simulink model "Bicycle_model"  (R2020a)
settings: Solver=VariableStepAuto  StartTime=0.0  StopTime=10.0  RelTol=1e-3
settings Model: Creator=yafta  LastModifiedBy=yafta

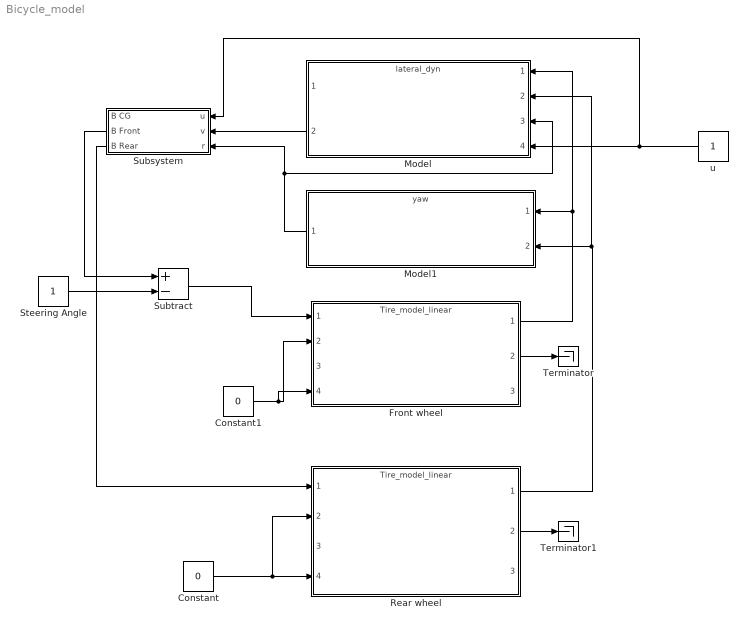
== system Bicycle_model ==
  Constant : Constant  Value=0
  Constant1 : Constant  Value=0
  Front wheel : ModelReference  ModelNameDialog=Tire_model_linear  SimulationMode=Normal  ModelReferenceVersion=1.2
  Model : ModelReference  ModelNameDialog=lateral_dyn.slx  SimulationMode=Normal  ModelReferenceVersion=1.2
  Model1 : ModelReference  ModelNameDialog=yaw.slx  SimulationMode=Normal  ModelReferenceVersion=1.1
  Rear wheel : ModelReference  ModelNameDialog=Tire_model_linear  SimulationMode=Normal  ModelReferenceVersion=1.2
  Steering Angle : Constant
  Subsystem : Subsystem
  Subtract : Sum  Inputs=+-
  Terminator : Terminator
  Terminator1 : Terminator
  u : Constant
  wires:
  Constant/1 -> Rear wheel/4, Rear wheel/2
  Constant1/1 -> Front wheel/4, Front wheel/2
  Front wheel/2 -> Terminator/1
  Rear wheel/2 -> Terminator1/1
  Rear wheel/1 -> Model/2, Model1/2
  Model1/1 -> Subsystem/3(r), Model/3
  Front wheel/1 -> Model/1, Model1/1
  Model/2 -> Subsystem/2(v)
  u/1 -> Subsystem/1(u), Model/4
  Subsystem/2(B Front) -> Subtract/1
  Steering Angle/1 -> Subtract/2
  Subtract/1 -> Front wheel/1
  Subsystem/3(B Rear) -> Rear wheel/1

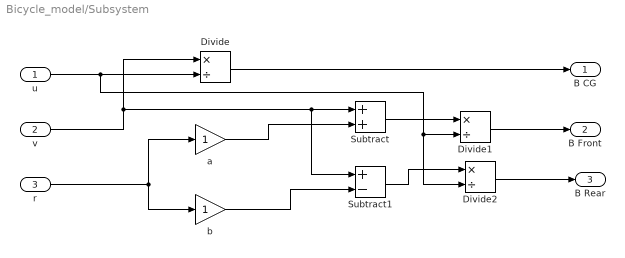
== system Bicycle_model/Subsystem ==
  u : Inport
  v : Inport  Port=2
  r : Inport  Port=3
  Divide : Product  Inputs=*/
  Divide1 : Product  Inputs=*/
  Divide2 : Product  Inputs=*/
  Subtract : Sum
  Subtract1 : Sum  Inputs=+-
  a : Gain
  b : Gain
  B CG : Outport
  B Front : Outport  Port=2
  B Rear : Outport  Port=3
  wires:
  v/1 -> Subtract1/1, Subtract/1, Divide/1
  u/1 -> Divide2/2, Divide1/2, Divide/2
  Divide/1 -> B CG/1
  r/1 -> a/1, b/1
  a/1 -> Subtract/2
  b/1 -> Subtract1/2
  Subtract/1 -> Divide1/1
  Subtract1/1 -> Divide2/1
  Divide1/1 -> B Front/1
  Divide2/1 -> B Rear/1
